simulink model "IC_Project_SimController"  (R2021b)
settings: Solver=VariableStepAuto  StartTime=0.0  StopTime=11.4  RelTol=1e-3
values from neighbouring files (symbols this model uses):
  A = [0,1;0,(1/m)*(p2+2*p3*vavg)]    [IC_Project_Observer_new.m]
  B = [0;p1/m]    [IC_Project_Observer_new.m]
  C = [0 1]    [IC_Project_Observer_new.m]
  ki = (0.46*tau + 0.02*T)/(Kpi*tau^2)    (= 0.562276785714)    [IC_Project_Controller_new.m]
  kp = (0.15*tau+0.35*T)/(Kpi*tau)    (= 2.22901785714)    [IC_Project_Controller_new.m]
settings Model: Creator=ethan  LastModifiedBy=ethan

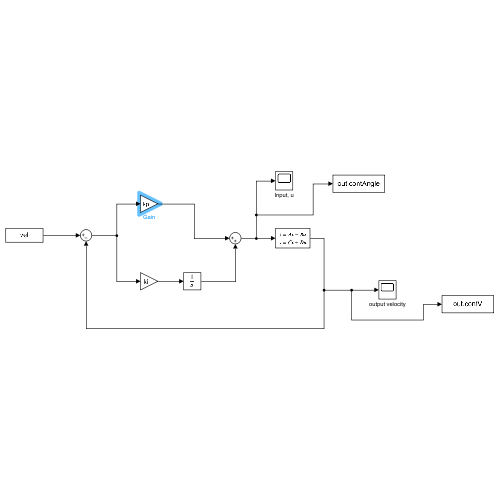
[thumbnail: Simulink's stored preview of the top-level diagram]
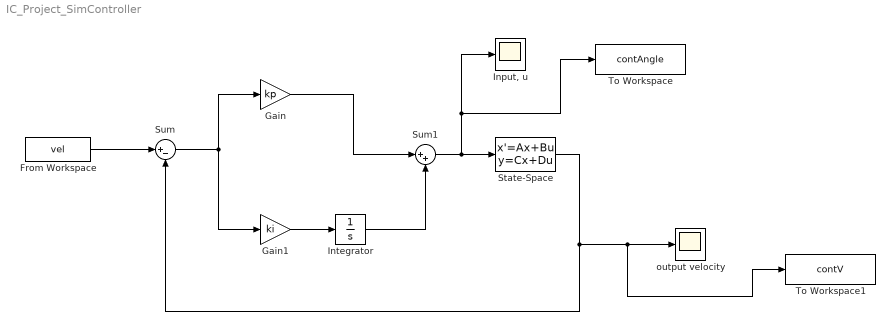
== system IC_Project_SimController ==
  From Workspace : FromWorkspace  VariableName=vel
  Gain : Gain  Gain=kp
  Gain1 : Gain  Gain=ki
  "Input, u" : Scope
  Integrator : Integrator
  State-Space : StateSpace  A=A  B=B  C=C  D=0  InitialCondition=0
  Sum : Sum  Inputs=|+-
  Sum1 : Sum  Inputs=|++
  To Workspace : ToWorkspace  VariableName=contAngle  SaveFormat=Timeseries  SampleTime=-1
  To Workspace1 : ToWorkspace  VariableName=contV  SaveFormat=Timeseries  SampleTime=-1
  output velocity : Scope
  wires:
  Sum/1 -> Gain1/1, Gain/1
  Gain1/1 -> Integrator/1
  Gain/1 -> Sum1/1
  Integrator/1 -> Sum1/2
  From Workspace/1 -> Sum/1
  State-Space/1 -> To Workspace1/1, output velocity/1, Sum/2
  Sum1/1 -> To Workspace/1, "Input, u"/1, State-Space/1
